simulink model "Block_Diagram"  (R2023a)
settings: Solver=VariableStepAuto  StartTime=0.0  StopTime=1  RelTol=1e-3
settings Model: Creator=Anirvan Krishna  LastModifiedBy=Anirvan Krishna
settings DataIOCC: Refine=500

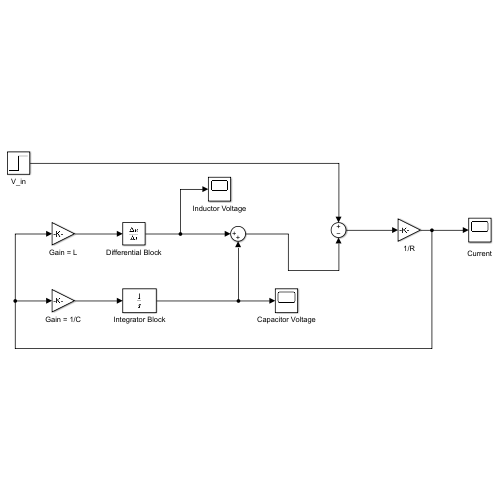
[thumbnail: Simulink's stored preview of the top-level diagram]
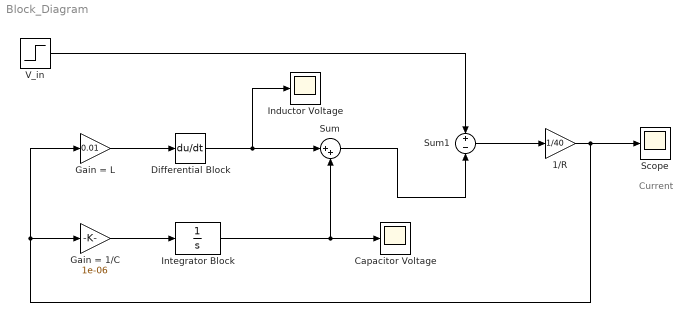
== system Block_Diagram ==
  note: Current
  1/R : Gain  Gain=1/40
  Capacitor Voltage : Scope
  Differential Block : Derivative
  Gain = 1/C : Gain  Gain=1e-06
  Gain = L : Gain  Gain=0.01
  Inductor Voltage : Scope
  Integrator Block : TransferFcn  Denominator=[1 0]
  Scope : Scope
  Sum : Sum  Inputs=|++
  Sum1 : Sum  Inputs=+-
  V_in : Step  Time=0.1  SampleTime=0
  wires:
  Differential Block/1 -> Inductor Voltage/1, Sum/1
  Gain = L/1 -> Differential Block/1
  Gain = 1/C/1 -> Integrator Block/1
  Integrator Block/1 -> Capacitor Voltage/1, Sum/2
  Sum/1 -> Sum1/2
  V_in/1 -> Sum1/1
  Sum1/1 -> 1/R/1
  1/R/1 -> Gain = 1/C/1, Gain = L/1, Scope/1
